simulink model "simulinkModel"  (R2021a)
settings: Solver=VariableStepAuto  StartTime=0.0  StopTime=3  RelTol=1e-3
libraries: audiosources x2, commutil2 x2, dspquant2 x2, commsrccod2 x1, dsparch4 x1, dspsigops x1
settings Model: Creator=Rohan  LastModifiedBy=Rohan

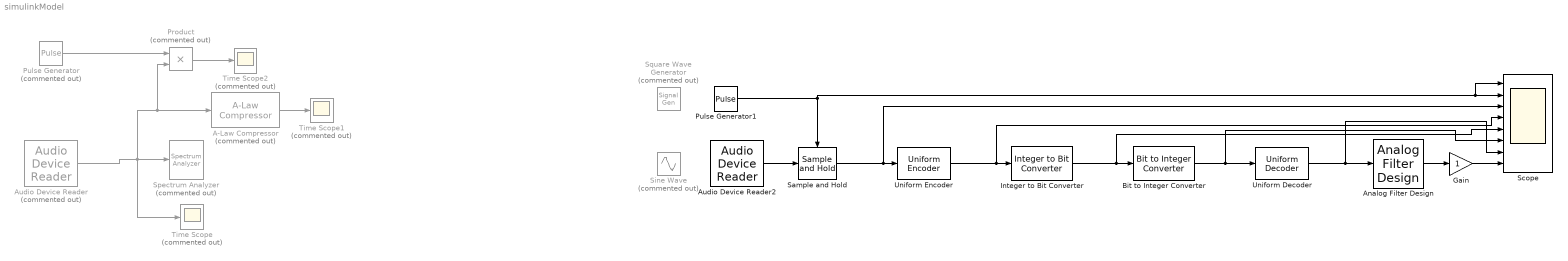
== system simulinkModel ==
  A-Law Compressor : commsrccod2/A-Law Compressor  Commented=on  A=87.6  V=1
      settings: SourceProductBaseCode=CM
  Analog Filter Design : dsparch4/Analog Filter Design  method=Butterworth  filttype=Lowpass  N=8  Wlo=2*pi*10  Whi=80  Rp=2  Rs=40
  Audio Device Reader : audiosources/Audio Device Reader  Commented=on  Driver=DirectSound  Device=Microphone Array (Realtek(R) Audio)  SampleRate=8000  NumChannels=1  SamplesPerFrame=1024  BitDepth=16-bit integer  NumBuffers=10  DefaultInputChannelMapping=on  InputChannelMapping=1:2  OutputNumOverrunSamples=off  OutputDataType=double  DriverIdx=1  DeviceWarnFlag=''
      settings: SourceProductBaseCode=AU
  Audio Device Reader2 : audiosources/Audio Device Reader  Driver=DirectSound  Device=Default  SampleRate=8000  NumChannels=1  SamplesPerFrame=1024  BitDepth=16-bit integer  NumBuffers=10  DefaultInputChannelMapping=on  InputChannelMapping=1:2  OutputNumOverrunSamples=off  OutputDataType=double  DriverIdx=1  DeviceWarnFlag=''
      settings: SourceProductBaseCode=AU
  Bit to Integer Converter : commutil2/Bit to Integer Converter  nbits=4  bitOrder=MSB first  signedOutputValues=Signed  outDtype=Inherit via internal rule  outDtypeSigned=Inherit via internal rule
  Gain : Gain
  Integer to Bit Converter : commutil2/Integer to Bit Converter  nbits=4  signedInputValues=Signed  bitOrder=MSB first  outDtype=Inherit via internal rule
  Product : Product  Commented=on
  Pulse Generator : DiscretePulseGenerator  Commented=on  PulseType=Time based  Period=10  PulseWidth=5
  Pulse Generator1 : DiscretePulseGenerator  PulseType=Time based  Amplitude=10  Period=1/100  PulseWidth=50
  Sample and Hold : dspsigops/Sample and Hold  trig=Rising edge  initCond=0  latchinput=off
  Scope : Scope  NumInputPorts=8
  Sine Wave : Sin  Commented=on  Amplitude=6  Frequency=2*pi*5  SampleTime=0
  Spectrum Analyzer : SpectrumAnalyzer  Commented=on
  Square Wave Generator : SignalGenerator  Commented=on  WaveForm=square  Amplitude=5  Frequency=5
  Time Scope : Scope  Commented=on
  Time Scope1 : Scope  Commented=on
  Time Scope2 : Scope  Commented=on
  Uniform Decoder : dspquant2/Uniform Decoder  peak=5  bits=4  overflowMode=Saturate  otype=Double
      settings: SourceProductBaseCode=DS
  Uniform Encoder : dspquant2/Uniform Encoder  peak=5  bits=4  otype=Signed integer
  wires:
  Audio Device Reader/1 -> Product/2, A-Law Compressor/1, Time Scope/1, Spectrum Analyzer/1
  A-Law Compressor/1 -> Time Scope1/1
  Pulse Generator/1 -> Product/1
  Product/1 -> Time Scope2/1
  Sample and Hold/1 -> Scope/3, Uniform Encoder/1
  Pulse Generator1/1 -> Scope/1, Scope/2, Sample and Hold/Trigger
  Uniform Encoder/1 -> Scope/4, Integer to Bit Converter/1
  Integer to Bit Converter/1 -> Scope/5, Bit to Integer Converter/1
  Bit to Integer Converter/1 -> Scope/6, Uniform Decoder/1
  Uniform Decoder/1 -> Analog Filter Design/1, Scope/7
  Analog Filter Design/1 -> Gain/1
  Gain/1 -> Scope/8
  Audio Device Reader2/1 -> Sample and Hold/1
